simulink model "scCO2_plant"  (R2024a)
settings: Solver=ode4  StartTime=0.0  StopTime=7200  FixedStep=0.1  RelTol=1e-3
libraries: slpidlib x1
settings Model: Creator=Vijai Venkatesh  LastModifiedBy=Vijai Venkatesh

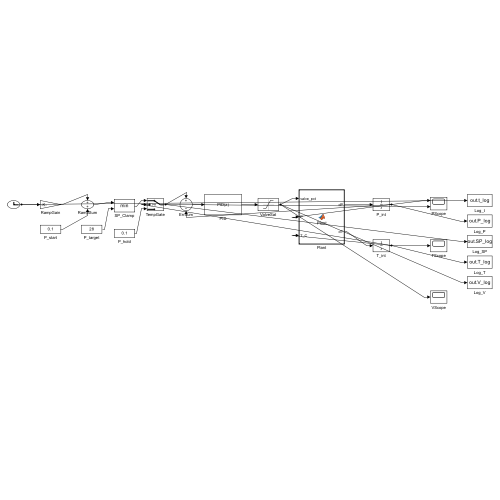
[thumbnail: Simulink's stored preview of the top-level diagram]
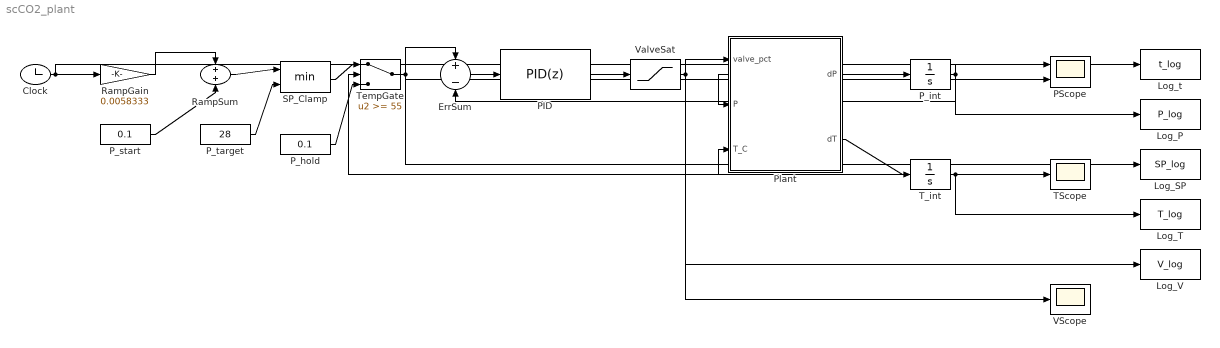
== system scCO2_plant ==
  Clock : Clock
  ErrSum : Sum  Inputs=+-
  Log_P : ToWorkspace  VariableName=P_log  SampleTime=0.1
  Log_SP : ToWorkspace  VariableName=SP_log  SampleTime=0.1
  Log_T : ToWorkspace  VariableName=T_log  SampleTime=0.1
  Log_V : ToWorkspace  VariableName=V_log  SampleTime=0.1
  Log_t : ToWorkspace  VariableName=t_log  SampleTime=0.1
  PID : slpidlib/PID Controller  Controller=PID  Form=Parallel  TimeDomain=Discrete-time  UseExternalTs=off  SampleTime=0.1  IntegratorMethod=Forward Euler  FilterMethod=Forward Euler  ControllerParametersSource=internal  P=40  I=5  UseKiTs=off  D=2  UseExternalDerivativeSource=off  N=20  UseFilter=on  TunerSelectOption=Transfer Function Based (PID Tuner App)  InitialConditionSource=internal  InitialConditionForIntegrator=0  InitialConditionForFilter=0  DifferentiatorICPrevScaledInput=0  ExternalReset=none  TrackingMode=off  Kt=1  LimitOutput=off  SatLimitsSource=internal  UpperSaturationLimit=100  LowerSaturationLimit=0  LinearizeAsGain=on  AntiWindupMode=clamping  Kb=1  LimitIntegrator=off  UpperIntegratorSaturationLimit=inf  LowerIntegratorSaturationLimit=-inf  POutMin=[]  POutMax=[]  IOutMin=[]  IOutMax=[]  DOutMin=[]  DOutMax=[]  NOutMin=[]  NOutMax=[]  SumOutMin=[]  SumOutMax=[]  SaturationOutMin=[]  SaturationOutMax=[]  PParamMin=[]  PParamMax=[]  IParamMin=[]  IParamMax=[]  DParamMin=[]  DParamMax=[]  NParamMin=[]  NParamMax=[]  KbParamMin=[]  KbParamMax=[]  KtParamMin=[]  KtParamMax=[]  KbOutMin=[]  KbOutMax=[]  KtOutMin=[]  KtOutMax=[]  IntegratorOutMin=[]  IntegratorOutMax=[]  FilterOutMin=[]  FilterOutMax=[]  SumI1OutMin=[]  SumI1OutMax=[]  SumI2OutMin=[]  SumI2OutMax=[]  SumI3OutMin=[]  SumI3OutMax=[]  SumI4OutMin=[]  SumI4OutMax=[]  SumDOutMin=[]  SumDOutMax=[]  DifferentiatorOutMin=[]  DifferentiatorOutMax=[]  FilterDiffOutCoefMin=[]  FilterDiffOutCoefMax=[]  ReciprocalOutMin=[]  ReciprocalOutMax=[]  SumDenOutMin=[]  SumDenOutMax=[]  SumNumOutMin=[]  SumNumOutMax=[]  DivideOutMin=[]  DivideOutMax=[]  UdiffTsProdOutMin=[]  UdiffTsProdOutMax=[]  NTsProdOutMin=[]  NTsProdOutMax=[]  UintegralTsProdOutMin=[]  UintegralTsProdOutMax=[]  UngainTsProdOutMin=[]  UngainTsProdOutMax=[]  ClampingZeroOutDataTypeStr=Inherit: Inherit via back propagation  ClampingZeroOutMin=[]  ClampingZeroOutMax=[]  FilterDenConstantOutDataTypeStr=Inherit: Inherit via back propagation  FilterDenConstantOutMin=[]  FilterDenConstantOutMax=[]  PCopyOutDataTypeStr=Inherit: Inherit via back propagation  PCopyOutMin=[]  PCopyOutMax=[]  NCopyOutDataTypeStr=Inherit: Inherit via back propagation  NCopyOutMin=[]  NCopyOutMax=[]  IntegratorContinuousStateAttributes=''  IntegratorStateMustResolveToSignalObject=off  IntegratorRTWStateStorageClass=Auto  FilterContinuousStateAttributes=''  FilterStateMustResolveToSignalObject=off  FilterRTWStateStorageClass=Auto  ParallelPVariant=InternalParameters  IdealPVariant=Disabled  IVariant=InternalParameters  DVariant=InternalParameters  IntegratorVariant=Discrete  SatVariant=Disabled  AWVariant=Passthrough  PCopyVariant=Disabled  TRVariant=Disabled  FdbkBlocksVariant=Forward  IdealPFdbkVariant=Disabled  SatFdbkVariant=Disabled  DerivativeFilterVariant=ForwardEulerFilter  NVariant=InternalParameters  NCopyVariant=Disabled  FilterICVariant=InternalICsFilter  IntegratorICVariant=InternalICs  ExternalResetVariant=Disabled  TRSumVariant=Passthrough  SumFdbkVariant=Disabled  SumVariant=Sum_PID  TsampFilterVariant=InternalTs  TsampNgainVariant=Passthrough  TsampIntegralVariant=Disabled_SignalSpec  ExternalSaturationOutDataTypeStr=Inherit: Same as second input  DerivativeSourceVariant=ErrorSignal
  PScope : Scope  NumInputPorts=2
  P_hold : Constant  Value=0.1
  P_int : Integrator  InitialCondition=0.1
  P_start : Constant  Value=0.1
  P_target : Constant  Value=28
  Plant : MATLAB Function  TreatAsAtomicUnit=on
  RampGain : Gain  Gain=0.0058333
  RampSum : Sum
  SP_Clamp : MinMax  Inputs=2
  TScope : Scope
  T_int : Integrator  InitialCondition=25
  TempGate : Switch  Threshold=55  SaturateOnIntegerOverflow=off  InputSameDT=off
  VScope : Scope
  ValveSat : Saturate  UpperLimit=100  LowerLimit=0
  wires:
  Clock/1 -> RampGain/1, Log_t/1
  RampGain/1 -> RampSum/1
  P_start/1 -> RampSum/2
  RampSum/1 -> SP_Clamp/1
  P_target/1 -> SP_Clamp/2
  SP_Clamp/1 -> TempGate/1
  T_int/1 -> TempGate/2, Plant/3(T_C), TScope/1, Log_T/1
  P_hold/1 -> TempGate/3
  TempGate/1 -> ErrSum/1, PScope/2, Log_SP/1
  P_int/1 -> ErrSum/2, Plant/2(P), PScope/1, Log_P/1
  ErrSum/1 -> PID/1
  PID/1 -> ValveSat/1
  ValveSat/1 -> Plant/1(valve_pct), VScope/1, Log_V/1
  Plant/1(dP) -> P_int/1
  Plant/2(dT) -> T_int/1

== matlab function scCO2_plant/Plant ==
  data: valve_pct input; dP output; P input; T_C input; dT output
function [dP, dT] = Plant(valve_pct, P, T_C)
P_BOOSTER=28.000000; K_FLOW=0.003000; K_COMP=0.800000; K_INK=0.067000; T_SET=60.000000;
v = valve_pct / 100;
dP_flow = K_FLOW * v * sqrt(max(P_BOOSTER - P, 0));
dP = dP_flow;
dT = K_COMP * dP_flow / P_BOOSTER - K_INK * (T_C - T_SET);
